simulink model "bpsk_fec_model_01"  (R2013a)
settings: Solver=FixedStepDiscrete  SolverMode=SingleTasking  StartTime=0.0  StopTime=(1e4 + 49)/600  RelTol=1e-3
PreLoadFcn:
  | maxNumErrs = 100;
  | maxNumBits = 1e6;
  | EbNo = 4;
InitFcn:
  | ;
StartFcn:
  | ;
StopFcn:
  | ;
undefined symbols (not defined in the file): DiscIntNeverNeededParam
libraries: dsparch4 x3, commsynccomp2 x3, dspsigops x3, simulink x2, commcnvcod2 x2, dspquant2 x1, commchan3 x1, commrandsrc2 x1, commsink2 x1
PreSaveFcn:
  | ;
CloseFcn:
  | ;
settings Model: MinMaxOverflowLogging=MinMaxAndOverflow  Creator=The MathWorks Inc.  LastModifiedBy=lifesatrip
settings DataIOCC: SignalLoggingSaveFormat=ModelDataLogs  SignalLogging=off  SaveTime=off
settings OptimizationCC: InlineParams=on  ExpressionDepthLimit=2147483647  LocalBlockOutputs=off  InitFltsAndDblsToZero=on  OptimizeModelRefInitCode=on  LifeSpan=1
settings DebuggingCC: SaveWithParameterizedLinksMsg=none  SignalResolutionControl=TryResolveAllWithWarning  MultiTaskDSMMsg=warning  MultiTaskCondExecSysMsg=none  FcnCallInpInsideContextMsg=UseLocalSettings  StrictBusMsg=Warning
settings HardwareCC: ProdBitPerInt=16  ProdIntDivRoundTo=Floor  ProdEndianess=LittleEndian  ProdWordSize=16  ProdHWDeviceType=16-bit Generic  TargetEndianess=LittleEndian  TargetHWDeviceType=MATLAB Host  ProdEqTarget=off
settings RTWCC: SystemTargetFile=ert.tlc  TemplateMakefile=ert_default_tmf  Description=Real-Time Workshop Embedded Coder (no auto configuration)  GenerateReport=on  RetainRTWFile=on  ProcessScript=ert_make_rtw_hook  IncludeHyperlinkInReport=on  LaunchReport=on  IncludeERTFirstTime=on
settings CodeAppCC: CustomSymbolStrType=$N$R$M  InternalIdentifier=Classic
settings ERTTargetCC: TargetFcnLib=ansi_tfl_tmw.mat  SupportAbsoluteTime=off  MatFileLogging=on  ERTCustomFileTemplate=example_file_process.tlc

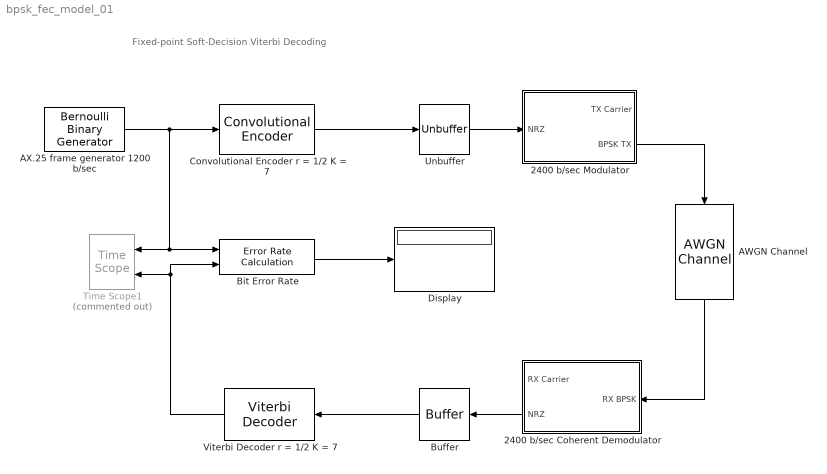
== system bpsk_fec_model_01 ==
  note: Fixed-point Soft-Decision Viterbi Decoding
  2400 b/sec Modulator : Subsystem
  2400 b/sec Coherent Demodulator : Subsystem
  AWGN Channel : commchan3/AWGN Channel  InputProcessing=Columns as channels (frame based)  seed=randseed  noiseMode="Signal to noise ratio  (Eb/No)"  EbNodB=inf  EsNodB=10  SNRdB=10  bitsPerSym=1  Ps=12.5  Tsym=1/2400  variance=1
  AX.25 frame generator 1200 b/sec : commrandsrc2/Bernoulli Binary Generator  P=0.5  seed=randseed  Ts=1/1200  frameBased=on  sampPerFrame=1  orient=off  outDataType=boolean
  Bit Error Rate : commsink2/Error Rate Calculation  N=50  st_delay=0  cp_mode=Entire frame  subframe=[]  PMode=Port  WsName=ErrorVec  RsMode2=off  stop=off  numErr=maxNumErrs  maxBits=maxNumBits
  Buffer : Buffer  N=2  TreatMby1Signals=One channel
  Convolutional Encoder r = 1/2 K = 7 : commcnvcod2/Convolutional Encoder  trellis=poly2trellis(7, [171 133])  opMode=Continuous  DelayedResetAction=off  hasIniStPort=off  hasFinStPort=off  usePuncVector=off  punctureVector=[1; 1; 0; 1; 0; 1]  reset=Unused parameter value
  Display : Display
      settings: Format=short_e
  Time Scope1 : TimeScope  Commented=on  NumInputPorts=2  DefaultConfigurationName=spbscopes.TimeScopeBlockCfg
      settings: CopyFcn=scopeextensions.ScopeBlock.callback(gcbh, 'onBlockCopy', gcbh);  DeleteFcn=scopeextensions.ScopeBlock.callback(gcbh, 'onBlockDelete');  PreSaveFcn=scopeextensions.ScopeBlock.callback(gcbh, 'onModelSave');  NameChangeFcn=scopeextensions.ScopeBlock.callback(gcbh, 'onBlockRename');  CloseFcn=scopeextensions.ScopeBlock.callback(gcbh, 'onBlockClose');  PreDeleteFcn=scopeextensions.ScopeBlock.callback(gcbh, 'onBlockPreDelete');
  Unbuffer : Unbuffer  SampleBasedProcessing=Same as frame based
  Viterbi Decoder r = 1/2 K = 7 : commcnvcod2/Viterbi Decoder  trellis=poly2trellis(7, [171 133])  isPunctured=off  punctureVector=[1; 1; 0; 1; 0; 1]  erasures=off  dectype=Soft decision  runSigValErrCheck=off  nsdecb=3  smWordLength=16  tbdepth=48  opmode=Continuous  reset=off  outDataType=boolean  delayedResetAction=off
  wires:
  Bit Error Rate/1 -> Display/1
  Viterbi Decoder r = 1/2 K = 7/1 -> Time Scope1/2, Bit Error Rate/2
  Convolutional Encoder r = 1/2 K = 7/1 -> Unbuffer/1
  Unbuffer/1 -> 2400 b/sec Modulator/1(NRZ)
  Buffer/1 -> Viterbi Decoder r = 1/2 K = 7/1
  2400 b/sec Coherent Demodulator/2(NRZ) -> Buffer/1
  2400 b/sec Modulator/2(BPSK TX) -> AWGN Channel/1
  AWGN Channel/1 -> 2400 b/sec Coherent Demodulator/1(RX BPSK)
  AX.25 frame generator 1200 b/sec/1 -> Convolutional Encoder r = 1/2 K = 7/1, Time Scope1/1, Bit Error Rate/1

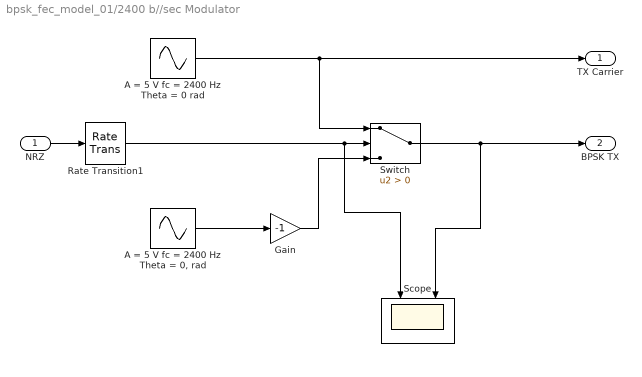
== system bpsk_fec_model_01/2400 b//sec Modulator ==
  NRZ : Inport
  A = 5 V fc = 2400 Hz Theta = 0 rad : Sin  Amplitude=5  Frequency=2*pi*4800  Phase=pi/2  SampleTime=1/480e3
  "A = 5 V fc = 2400 Hz Theta = 0, rad" : Sin  Amplitude=5  Frequency=2*pi*4800  Phase=pi/2  Samples=100  SampleTime=1/480e3  Offset=pi
  Gain : Gain  Gain=-1
  Rate Transition1 : RateTransition  OutPortSampleTime=1/480e3
  Scope : Scope  NumInputPorts=2
      settings: TimeRange=0.06  YMin=-1000~-0.5  YMax=1000~1.5  SaveName=ScopeData2
  Switch : Switch  Criteria=u2 > Threshold
  TX Carrier : Outport
  BPSK TX : Outport  Port=2
  wires:
  A = 5 V fc = 2400 Hz Theta = 0 rad/1 -> TX Carrier/1, Switch/1
  "A = 5 V fc = 2400 Hz Theta = 0, rad"/1 -> Gain/1
  Gain/1 -> Switch/3
  NRZ/1 -> Rate Transition1/1
  Switch/1 -> BPSK TX/1, Scope/2
  Rate Transition1/1 -> Scope/1, Switch/2

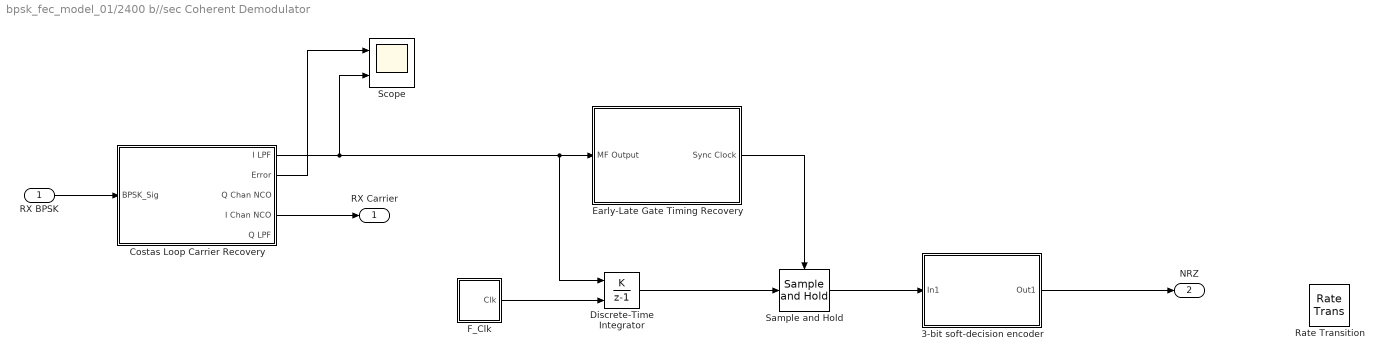
== system bpsk_fec_model_01/2400 b//sec Coherent Demodulator ==
  RX BPSK : Inport
  3-bit soft-decision encoder : Subsystem
  Costas Loop Carrier Recovery : Subsystem
  Discrete-Time Integrator : DiscreteIntegrator  IntegratorMethod=Accumulation: Forward Euler  ExternalReset=rising  SampleTime=1/480e3  ICPrevOutput=DiscIntNeverNeededParam  ICPrevScaledInput=DiscIntNeverNeededParam
  Early-Late Gate Timing Recovery : Subsystem
  F_Clk : Subsystem
  Rate Transition : RateTransition  OutPortSampleTime=1/1200
  Sample and Hold : dspsigops/Sample and Hold  trig=Rising edge  initCond=0  latchinput=off
  Scope : Scope  NumInputPorts=2
      settings: TimeRange=0.0403041825095057  YMin=-30~-12.5  YMax=30~12.5
  RX Carrier : Outport
  NRZ : Outport  Port=2
  wires:
  RX BPSK/1 -> Costas Loop Carrier Recovery/1(BPSK_Sig)
  Early-Late Gate Timing Recovery/1(Sync Clock) -> Sample and Hold/Trigger
  Costas Loop Carrier Recovery/1(I LPF) -> Scope/2, Discrete-Time Integrator/1, Early-Late Gate Timing Recovery/1(MF Output)
  Costas Loop Carrier Recovery/2(Error) -> Scope/1
  Discrete-Time Integrator/1 -> Sample and Hold/1
  F_Clk/1(Clk) -> Discrete-Time Integrator/2
  Costas Loop Carrier Recovery/4(I Chan NCO) -> RX Carrier/1
  Sample and Hold/1 -> 3-bit soft-decision encoder/1(In1)
  3-bit soft-decision encoder/1(Out1) -> NRZ/1

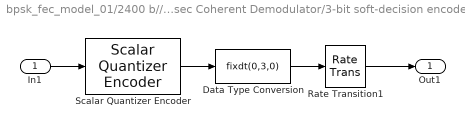
== system bpsk_fec_model_01/2400 b//sec Coherent Demodulator/3-bit soft-decision encoder ==
  In1 : Inport
  Data Type Conversion : DataTypeConversion  OutDataTypeStr=fixdt(0,3,0)
  Rate Transition1 : RateTransition  OutPortSampleTime=1/2400
  Scalar Quantizer Encoder : dspquant2/Scalar Quantizer Encoder  paramSrc=Specify via dialog  partType=Unbounded  BBoundary=[-250:250]  UBoundary=[-250 -167 -83 0 83 167 250]  SearchMethod=Linear  tieBreakRule=Choose the higher index  outQU=off  outQError=off  codebook=[1.5:9.5]  outStatus=off  invalidin=Clip  idtype=uint8  roundingMode=Floor  overflowMode=off
  Out1 : Outport
  wires:
  In1/1 -> Scalar Quantizer Encoder/1
  Scalar Quantizer Encoder/1 -> Data Type Conversion/1
  Data Type Conversion/1 -> Rate Transition1/1
  Rate Transition1/1 -> Out1/1

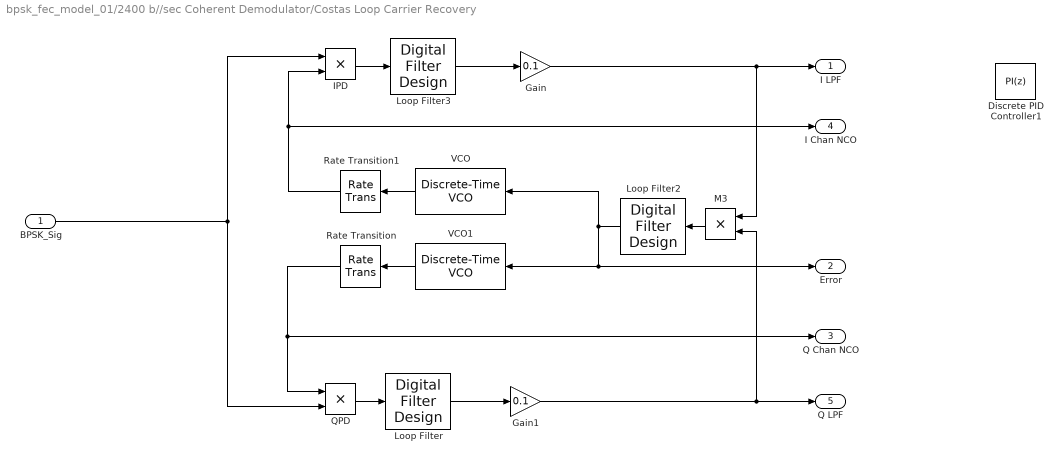
== system bpsk_fec_model_01/2400 b//sec Coherent Demodulator/Costas Loop Carrier Recovery ==
  BPSK_Sig : Inport
  Discrete PID Controller1 : simulink/Continuous/PID Controller  Controller=PI  TimeDomain=Discrete-time  SampleTime=1/480e3  IntegratorMethod=Forward Euler  FilterMethod=Forward Euler  Form=Parallel  P=0.05  I=0.00075  D=0  N=100  InitialConditionSource=internal  InitialConditionForIntegrator=0  InitialConditionForFilter=0  ExternalReset=none  LimitOutput=off  UpperSaturationLimit=inf  LowerSaturationLimit=-inf  LinearizeAsGain=off  AntiWindupMode=none  Kb=1  TrackingMode=off  Kt=1  PParamMin=[]  PParamMax=[]  IParamMin=[]  IParamMax=[]  DParamMin=[]  DParamMax=[]  NParamMin=[]  NParamMax=[]  KbParamMin=[]  KbParamMax=[]  KtParamMin=[]  KtParamMax=[]  POutMin=[]  POutMax=[]  IOutMin=[]  IOutMax=[]  DOutMin=[]  DOutMax=[]  NOutMin=[]  NOutMax=[]  KbOutMin=[]  KbOutMax=[]  KtOutMin=[]  KtOutMax=[]  IntegratorOutMin=[]  IntegratorOutMax=[]  FilterOutMin=[]  FilterOutMax=[]  SumOutMin=[]  SumOutMax=[]  SumI1OutMin=[]  SumI1OutMax=[]  SumI2OutMin=[]  SumI2OutMax=[]  SumI3OutMin=[]  SumI3OutMax=[]  SumDOutMin=[]  SumDOutMax=[]  SaturationOutMin=[]  SaturationOutMax=[]  IntegratorContinuousStateAttributes=''  IntegratorStateMustResolveToSignalObject=off  IntegratorRTWStateStorageClass=Auto  FilterContinuousStateAttributes=''  FilterStateMustResolveToSignalObject=off  FilterRTWStateStorageClass=Auto
  Gain : Gain  Gain=0.1
  Gain1 : Gain  Gain=0.1
  IPD : Product  SampleTime=1/480e3
  Loop Filter : dsparch4/Digital Filter Design  mwdsp_browser_bugfix_var=off
  Loop Filter2 : dsparch4/Digital Filter Design  mwdsp_browser_bugfix_var=off
  Loop Filter3 : dsparch4/Digital Filter Design  mwdsp_browser_bugfix_var=off
  M3 : Product  SampleTime=1/480e3
  QPD : Product  SampleTime=1/480e3
  Rate Transition : RateTransition  OutPortSampleTime=1/480e3
  Rate Transition1 : RateTransition  OutPortSampleTime=1/480e3
  VCO : commsynccomp2/Discrete-Time VCO  Ac=5  Fc=4800  Kc=0.5  Ph=0  ts=1/480e3
  VCO1 : commsynccomp2/Discrete-Time VCO  Ac=5  Fc=4800  Kc=0.5  Ph=pi/2  ts=1/480e3
  I LPF : Outport
  Error : Outport  Port=2
  Q Chan NCO : Outport  Port=3
  I Chan NCO : Outport  Port=4
  Q LPF : Outport  Port=5
  wires:
  VCO/1 -> Rate Transition1/1
  VCO1/1 -> Rate Transition/1
  Rate Transition/1 -> QPD/1, Q Chan NCO/1
  Rate Transition1/1 -> IPD/2, I Chan NCO/1
  QPD/1 -> Loop Filter/1
  IPD/1 -> Loop Filter3/1
  BPSK_Sig/1 -> IPD/1, QPD/2
  Loop Filter/1 -> Gain1/1
  Loop Filter3/1 -> Gain/1
  M3/1 -> Loop Filter2/1
  Loop Filter2/1 -> VCO/1, Error/1, VCO1/1
  Gain/1 -> I LPF/1, M3/1
  Gain1/1 -> Q LPF/1, M3/2

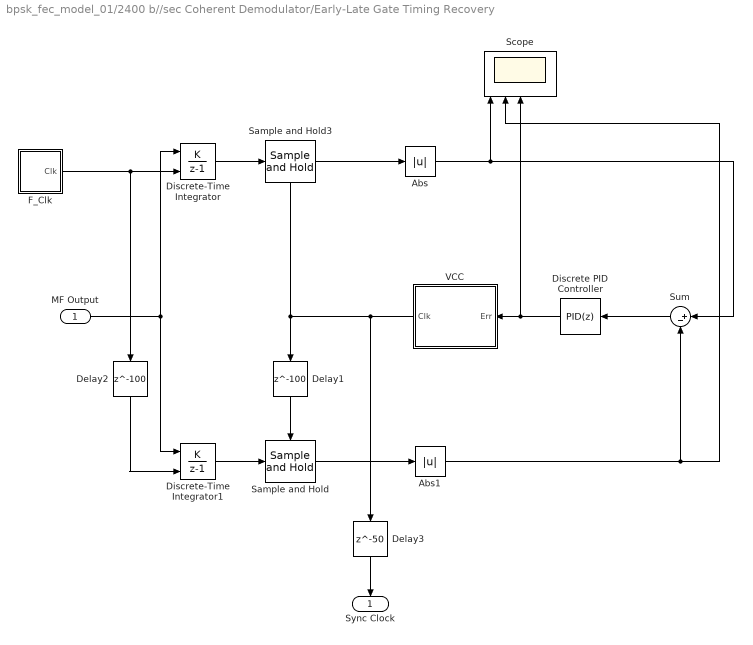
== system bpsk_fec_model_01/2400 b//sec Coherent Demodulator/Early-Late Gate Timing Recovery ==
  MF Output : Inport
  Abs : Abs
  Abs1 : Abs
  Delay1 : Delay  DelayLength=100  InitialCondition=0
  Delay2 : Delay  DelayLength=100  InitialCondition=0
  Delay3 : Delay  DelayLength=50  InitialCondition=0
  Discrete PID Controller : simulink/Continuous/PID Controller  Controller=PID  TimeDomain=Discrete-time  SampleTime=1/480e3  IntegratorMethod=Forward Euler  FilterMethod=Forward Euler  Form=Parallel  P=0.1  I=0.01  D=0  N=0  InitialConditionSource=internal  InitialConditionForIntegrator=0  InitialConditionForFilter=0  ExternalReset=none  LimitOutput=off  UpperSaturationLimit=inf  LowerSaturationLimit=-inf  LinearizeAsGain=off  AntiWindupMode=none  Kb=1  TrackingMode=off  Kt=1  PParamMin=[]  PParamMax=[]  IParamMin=[]  IParamMax=[]  DParamMin=[]  DParamMax=[]  NParamMin=[]  NParamMax=[]  KbParamMin=[]  KbParamMax=[]  KtParamMin=[]  KtParamMax=[]  POutMin=[]  POutMax=[]  IOutMin=[]  IOutMax=[]  DOutMin=[]  DOutMax=[]  NOutMin=[]  NOutMax=[]  KbOutMin=[]  KbOutMax=[]  KtOutMin=[]  KtOutMax=[]  IntegratorOutMin=[]  IntegratorOutMax=[]  FilterOutMin=[]  FilterOutMax=[]  SumOutMin=[]  SumOutMax=[]  SumI1OutMin=[]  SumI1OutMax=[]  SumI2OutMin=[]  SumI2OutMax=[]  SumI3OutMin=[]  SumI3OutMax=[]  SumDOutMin=[]  SumDOutMax=[]  SaturationOutMin=[]  SaturationOutMax=[]  IntegratorContinuousStateAttributes=''  IntegratorStateMustResolveToSignalObject=off  IntegratorRTWStateStorageClass=Auto  FilterContinuousStateAttributes=''  FilterStateMustResolveToSignalObject=off  FilterRTWStateStorageClass=Auto
  Discrete-Time Integrator : DiscreteIntegrator  IntegratorMethod=Accumulation: Forward Euler  ExternalReset=rising  SampleTime=1/480e3  ICPrevOutput=DiscIntNeverNeededParam  ICPrevScaledInput=DiscIntNeverNeededParam
  Discrete-Time Integrator1 : DiscreteIntegrator  IntegratorMethod=Accumulation: Forward Euler  ExternalReset=rising  SampleTime=1/480e3  ICPrevOutput=DiscIntNeverNeededParam  ICPrevScaledInput=DiscIntNeverNeededParam
  F_Clk : Subsystem
  Sample and Hold : dspsigops/Sample and Hold  trig=Rising edge  initCond=0  latchinput=off
  Sample and Hold3 : dspsigops/Sample and Hold  trig=Rising edge  initCond=0  latchinput=off
  Scope : Scope  NumInputPorts=5
      settings: TimeRange=0.06  YMin=110~115~-100~-0.5~-200  YMax=160~160~125~1.5~200  SaveName=ScopeData3
  Sum : Sum  Inputs=|+-
  VCC : Subsystem
  Sync Clock : Outport
  wires:
  Abs1/1 -> Scope/2, Sum/2
  Sample and Hold/1 -> Abs1/1
  Sample and Hold3/1 -> Abs/1
  Sum/1 -> Discrete PID Controller/1
  VCC/1(Clk) -> Delay3/1, Delay1/1, Sample and Hold3/Trigger
  MF Output/1 -> Discrete-Time Integrator/1, Discrete-Time Integrator1/1
  Discrete-Time Integrator/1 -> Sample and Hold3/1
  Discrete-Time Integrator1/1 -> Sample and Hold/1
  Delay2/1 -> Discrete-Time Integrator1/2
  Delay1/1 -> Sample and Hold/Trigger
  Delay3/1 -> Sync Clock/1
  F_Clk/1(Clk) -> Delay2/1, Discrete-Time Integrator/2
  Discrete PID Controller/1 -> Scope/3, VCC/1(Err)
  Abs/1 -> Sum/1, Scope/1

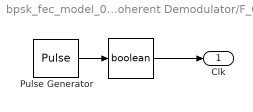
== system bpsk_fec_model_01/2400 b//sec Coherent Demodulator/F_Clk ==
  " " : DataTypeConversion  OutDataTypeStr=boolean
  Pulse Generator : DiscretePulseGenerator  PulseType=Time based  Amplitude=5  Period=1/2400  PulseWidth=50  SampleTime=1/480e3
  Clk : Outport
  wires:
  " "/1 -> Clk/1
  Pulse Generator/1 -> " "/1

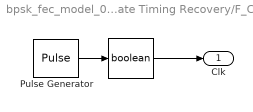
== system bpsk_fec_model_01/2400 b//sec Coherent Demodulator/Early-Late Gate Timing Recovery/F_Clk ==
  " " : DataTypeConversion  OutDataTypeStr=boolean
  Pulse Generator : DiscretePulseGenerator  PulseType=Time based  Amplitude=5  Period=1/2400  PulseWidth=50  SampleTime=1/480e3
  Clk : Outport
  wires:
  " "/1 -> Clk/1
  Pulse Generator/1 -> " "/1

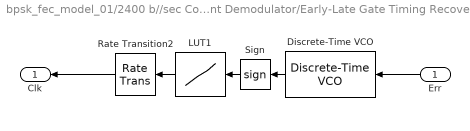
== system bpsk_fec_model_01/2400 b//sec Coherent Demodulator/Early-Late Gate Timing Recovery/VCC ==
  Err : Inport
  Discrete-Time VCO : commsynccomp2/Discrete-Time VCO  Ac=1  Fc=2400  Kc=1  Ph=0  ts=1/480e3
  LUT1 : Lookup_n-D  NumberOfTableDimensions=1  BreakpointsForDimension1=[-1 0 1]  Table=[0 0 1]  RndMeth=Simplest  InputSameDT=on
  Rate Transition2 : RateTransition  OutPortSampleTime=1/480e3
  Sign : Signum
  Clk : Outport
  wires:
  Discrete-Time VCO/1 -> Sign/1
  Err/1 -> Discrete-Time VCO/1
  LUT1/1 -> Rate Transition2/1
  Rate Transition2/1 -> Clk/1
  Sign/1 -> LUT1/1
